simulink model "ur3_simulink_ros2_ibvs_mpc"  (R2023b)
settings: Solver=ode4  StartTime=0.0  StopTime=Inf  FixedStep=0.005  RelTol=1e-3
model workspace (MAT data in the model file):
  SL_ROS_VariableLengthArrays_MaxSizes : object (value not decoded)
undefined symbols (not defined in the file): data, data_SL_Info
libraries: simulink x9, ros2lib x8, robotmaniplib x3, robotcorelib x2, dspinverses x1, mpclib x1
(part 2 of 2)

== matlab function ur3_simulink_ros2_ibvs_mpc/APO+AIC/Subsystem3/APO+AIC/MATLAB Function ==
  data: count output; hat_x_last input; predict_y_last input; y_real input; y2_derivative_sampling input; u_last input; delta_u_last input; hat_x output; t_now input; A_bar input; B_bar input; C_bar input; predict_y output; A0 input; B0 input; mu_last input; mu_p_last input; u output; delta_u output; mu output; mu_p output
function [count,hat_x,predict_y, u, delta_u, mu, mu_p] = fcn(hat_x_last, predict_y_last, y_real,y2_derivative_sampling, u_last,delta_u_last,t_now,A_bar,B_bar,C_bar,A0,B0,mu_last, mu_p_last)
if(t_now==0)
    count=0;
    hat_x = zeros(2,1);
    predict_y = y_real;
    hat_x(1,1)=y_real;
    [u, delta_u, mu, mu_p]  = AIC2(t_now, 1, y_real,hat_x(1,1),y2_derivative_sampling,hat_x(2,1), mu_last, mu_p_last, u_last);
else
    count=mod(t_now,0.05);
    if(count==0)%在采样的时刻
        predict_y=y_real;
        hat_x=A_bar*hat_x_last +B_bar*delta_u_last/0.01+ C_bar*predict_y;
        [u, delta_u, mu, mu_p]  = AIC2(t_now, 1, y_real,hat_x(1,1),y2_derivative_sampling,hat_x(2,1), mu_last, mu_p_last, u_last);
    else%在两个采样时刻之间
        predict_y=[1 0]*(A0*hat_x_last+B0*delta_u_last);
        hat_x=A_bar*hat_x_last + B_bar*delta_u_last/0.01+C_bar*predict_y_last;
        [u, delta_u, mu, mu_p]  = AIC2(t_now, 1, y_real,hat_x(1,1),y2_derivative_sampling,hat_x(2,1), mu_last, mu_p_last, u_last);
    end
end
end








% function [count,hat_x,predict_y, u, delta_u, mu, mu_p, mu_pp] = fcn(hat_x_last, predict_y_last, y_real,y2_derivative_sampling,y3_real_slow, u_last,delta_u_last,t_now,A_bar,B_bar,C_bar,A0,B0,mu_last, mu_p_last, mu_pp_last)
% if(t_now==0)
%     count=0;
%     hat_x = zeros(3,1);
%     predict_y = y_real;
%     hat_x(1,1)=y_real;
%     u_now=0;
%     hat_x = A_bar*hat_x + B_bar*u_now+ C_bar*predict_y;
%     [u, delta_u, mu, mu_p, mu_pp]  = AIC3(t_now, 1, y_real,hat_x(1,1),y2_derivative_sampling,hat_x(2,1), y3_real_slow, hat_x(3,1), mu_last, mu_p_last, mu_pp_last, u_last);
%     %predict_y=[1 0 0]*(A0*hat_x+B0*delta_u); 
%     
% else
%     count=mod(t_now,0.05);
%     if(count==0)%在采样的时刻
%         predict_y=y_real;
%         hat_x=A_bar*hat_x_last +B_bar*delta_u_last+ C_bar*predict_y;
%         %hat_x(1,1)=y_real;
%         [u, delta_u, mu, mu_p, mu_pp]  = AIC3(t_now, 1, y_real,hat_x(1,1),y2_derivative_sampling,hat_x(2,1), y3_real_slow, hat_x(3,1), mu_last, mu_p_last, mu_pp_last, u_last);
% 
%         %predict_y=[1 0 0]*(A0*hat_x+B0*delta_u);
%         
%     else%在两个采样时刻之间
%         predict_y=[1 0 0]*(A0*hat_x_last+B0*delta_u_last);
%         hat_x=A_bar*hat_x_last + B_bar*delta_u_last+C_bar*predict_y_last;
%         [u, delta_u, mu, mu_p, mu_pp]  = AIC3(t_now, 1, y_real,hat_x(1,1),y2_derivative_sampling,hat_x(2,1), y3_real_slow, hat_x(3,1), mu_last, mu_p_last, mu_pp_last, u_last);
%         %predict_y=[1 0 0]*(A0*hat_x+B0*delta_u);
%         
%     end
% end
% end

== matlab function ur3_simulink_ros2_ibvs_mpc/AIC/Subsystem1/AIC_muti_sensor_module/MATLAB Function ==
  data: u output; y1_real_slow input; y2_derivative_sampling input; mu output; mu_p output; mu_last input; mu_p_last input; u_last input
function [u, mu, mu_p]  = fcn(y1_real_slow,y2_derivative_sampling, mu_last, mu_p_last, u_last)
e_1=2;
e_2=2;
k_l=1;
sigma_z1_inv=0.2;
sigma_z2_inv=0.2;
sigma_w1_inv=1;
sigma_w2_inv=1;
k_i=1.2;
k_p=2.4;
T_c=0.05;
mu = double(mu_last + T_c*(mu_p_last+k_l*sigma_z1_inv*(y1_real_slow-mu_last)-k_l*sigma_w1_inv*e_1*(mu_p_last+e_1*mu_last)));
mu_p = double(mu_p_last + T_c*(k_l*sigma_z2_inv*(y2_derivative_sampling-mu_p_last)-k_l*sigma_w1_inv*(mu_p_last+e_1*mu_last)-k_l*sigma_w2_inv*e_2*e_2*mu_p_last));
u = double( u_last - T_c*(k_i*(y1_real_slow-mu)+k_p*(y2_derivative_sampling-mu_p)));
end

== matlab function ur3_simulink_ros2_ibvs_mpc/AIC/Subsystem2/AIC_muti_sensor_module/MATLAB Function ==
  data: u output; y1_real_slow input; y2_derivative_sampling input; mu output; mu_p output; mu_last input; mu_p_last input; u_last input
function [u, mu, mu_p]  = fcn(y1_real_slow,y2_derivative_sampling, mu_last, mu_p_last, u_last)
e_1=2;
e_2=2;
k_l=1;
sigma_z1_inv=0.2;
sigma_z2_inv=0.2;
sigma_w1_inv=1;
sigma_w2_inv=1;
k_i=1.2;
k_p=2.4;
T_c=0.05;
mu = double(mu_last + T_c*(mu_p_last+k_l*sigma_z1_inv*(y1_real_slow-mu_last)-k_l*sigma_w1_inv*e_1*(mu_p_last+e_1*mu_last)));
mu_p = double(mu_p_last + T_c*(k_l*sigma_z2_inv*(y2_derivative_sampling-mu_p_last)-k_l*sigma_w1_inv*(mu_p_last+e_1*mu_last)-k_l*sigma_w2_inv*e_2*e_2*mu_p_last));
u = double( u_last - T_c*(k_i*(y1_real_slow-mu)+k_p*(y2_derivative_sampling-mu_p)));
end

== matlab function ur3_simulink_ros2_ibvs_mpc/AIC/Subsystem3/AIC_muti_sensor_module/MATLAB Function ==
  data: u output; y1_real_slow input; y2_derivative_sampling input; mu output; mu_p output; mu_last input; mu_p_last input; u_last input
function [u, mu, mu_p]  = fcn(y1_real_slow,y2_derivative_sampling, mu_last, mu_p_last, u_last)
e_1=2;
e_2=2;
k_l=1;
sigma_z1_inv=0.2;
sigma_z2_inv=0.2;
sigma_w1_inv=1;
sigma_w2_inv=1;
k_i=1.2;
k_p=2.4;
T_c=0.05;
mu = double(mu_last + T_c*(mu_p_last+k_l*sigma_z1_inv*(y1_real_slow-mu_last)-k_l*sigma_w1_inv*e_1*(mu_p_last+e_1*mu_last)));
mu_p = double(mu_p_last + T_c*(k_l*sigma_z2_inv*(y2_derivative_sampling-mu_p_last)-k_l*sigma_w1_inv*(mu_p_last+e_1*mu_last)-k_l*sigma_w2_inv*e_2*e_2*mu_p_last));
u = double( u_last - T_c*(k_i*(y1_real_slow-mu)+k_p*(y2_derivative_sampling-mu_p)));
end

== matlab function ur3_simulink_ros2_ibvs_mpc/Subsystem1/Subsystem/MATLAB Function ==
  data: u input; u1 output; v1 output; u2 output; v2 output; u3 output; v3 output; u4 output; v4 output
function [u1,v1,u2,v2,u3,v3,u4,v4] = fcn(u)
u1 = u(1);
v1 = u(2);
u2 = u(3);
v2 = u(4);
u3 = u(5);
v3 = u(6);
u4 = u(7);
v4 = u(8);

== matlab function ur3_simulink_ros2_ibvs_mpc/ROS2 Time Generator/MATLAB Function ==
  data: current_time input; last_time input; time_x output; init_time output
function [time_x,init_time] = fcn(current_time, last_time)
init_time = last_time;
time_x = current_time-last_time;

== matlab function ur3_simulink_ros2_ibvs_mpc/Subsystem2/dob for ibvs ==
  data: last_d_temp input size=8; x input size=8; last_x input size=8; b input size=[8,6]; u input size=6; d output size=11; l_gain input; d_temp output size=8; Ts input
function [d,d_temp] = fcn(last_d_temp,x,last_x,b,u,l_gain,Ts)
d_temp = last_d_temp - Ts*l_gain*last_d_temp + l_gain*(x-last_x-Ts*b*u);
d = [d_temp;0;0;0];

== matlab function ur3_simulink_ros2_ibvs_mpc/Subsystem/MATLAB Function ==
  data: u input; y output
function y = fcn(u)
y = zeros(1,128);
y(1) = u;
y(2) = u;
y(3) = u;
y(4) = -u;
y(5) = -u;
y(6) = -u;
y(7) = -u;
y(8) = u;

== matlab function ur3_simulink_ros2_ibvs_mpc/MATLAB Function1 ==
  data: refer input; pixel_error output; real input
function pixel_error = fcn(refer,real)
pixel_error = zeros(8,1);
pixel_error(1) = refer(1) -real(1);
pixel_error(2) = refer(2) -real(2);
pixel_error(3) = refer(3) -real(3);
pixel_error(4) = refer(4) -real(4);
pixel_error(5) = refer(5) -real(5);
pixel_error(6) = refer(6) -real(6);
pixel_error(7) = refer(7) -real(7);
pixel_error(8) = refer(8) -real(8);

== matlab function ur3_simulink_ros2_ibvs_mpc/Subsystem4/model refresher/state fuction ==
  data: pixel input; ee_position input; A output; U_in input; ee_jacobian input; B output; C output; D output; U output; Y output; X output; DX output; new_jacobian input; mix_jacobian output
function [A, B, C, D, U, Y, X, DX,mix_jacobian] = fcn(pixel,ee_position, U_in, ee_jacobian, new_jacobian)
A = zeros(11,11);
C = eye(11);
D = zeros(11,17);
X=[pixel;ee_position];
[B,mix_jacobian] = getContinuous(X,ee_jacobian,new_jacobian);
U=U_in;
DZ = B*U_in;
DX = [DZ(1);DZ(2);DZ(3);DZ(4);DZ(5);DZ(6);DZ(7);DZ(8);DZ(9);DZ(10);DZ(11)];
Y=X;

function  [b,mix_jacobian] = getContinuous(x,k_jacobian,newk_jacobian)
b = zeros(11, 17);
% states
u_1 = x(1);
v_1 = x(2);
u_2 = x(3);
v_2 = x(4);
u_3 = x(5);
v_3 = x(6);
u_4 = x(7);
v_4 = x(8);
% parameters
f = 900;            %focal length of realsenseD455=1930um
p_size = 0;        %Pixel Size of realsenseD4455=3um
f_pixel = 900;       %the focal length in pixels f/p_size
Z = 0.25;             %Depth estimate for four points
% image jcobian
i_jcobian = [-f_pixel/Z,0,u_1/Z,u_1*v_1/f_pixel,-(f_pixel^2+u_1^2)/f_pixel,v_1;
             0,-f_pixel/Z,v_1/Z,(f_pixel^2+v_1^2)/f_pixel,-u_1*v_1/f_pixel,-u_1;
             -f_pixel/Z,0,u_2/Z,u_2*v_2/f_pixel,-(f_pixel^2+u_2^2)/f_pixel,v_2;
             0,-f_pixel/Z,v_2/Z,(f_pixel^2+v_2^2)/f_pixel,-u_2*v_2/f_pixel,-u_2;
             -f_pixel/Z,0,u_3/Z,u_3*v_3/f_pixel,-(f_pixel^2+u_3^2)/f_pixel,v_3;
             0,-f_pixel/Z,v_3/Z,(f_pixel^2+v_3^2)/f_pixel,-u_3*v_3/f_pixel,-u_3;
             -f_pixel/Z,0,u_4/Z,u_4*v_4/f_pixel,-(f_pixel^2+u_4^2)/f_pixel,v_4;
             0,-f_pixel/Z,v_4/Z,(f_pixel^2+v_4^2)/f_pixel,-u_4*v_4/f_pixel,-u_4];
mix_jacobian = i_jcobian*newk_jacobian;
disturbance_mat = zeros(11, 11);
disturbance_mat(1:8, 1:8) = eye(8);
% state equations
b(1:8, 1:6) = mix_jacobian;
b(9:11, 1:6) = k_jacobian(1:3,1:6);
b(1:11, 7:17) = disturbance_mat;
